simulink library "notificaStato"  (R2024b)
settings: Solver=VariableStepAuto  StartTime=0.0  StopTime=10.0  RelTol=1e-3
settings Model: Creator=mainuser  LastModifiedBy=mainuser

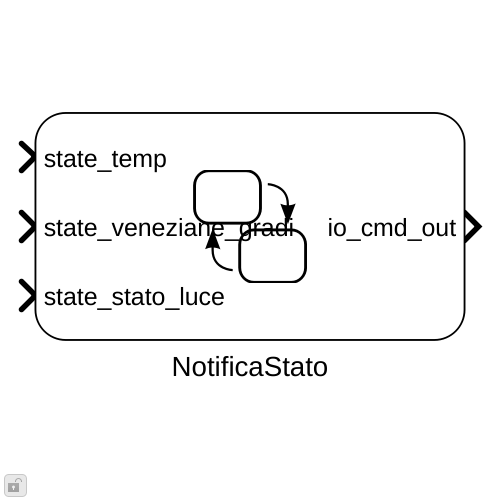
[thumbnail: Simulink's stored preview of the top-level diagram]
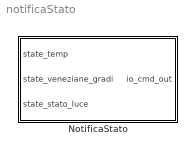
== system notificaStato ==
  NotificaStato : Stateflow chart  TreatAsAtomicUnit=on

== stateflow chart notificaStato/NotificaStato ==
  state SendNotify
    en: io_cmd_out = send_notifica(...
    state_temp, ...
    state_veneziane_gradi, ...
    state_stato_luce...
    )
  state Wait
  (default) -> SendNotify
  SendNotify -> Wait
  Wait -> SendNotify : after(10,sec)
  data: temp function_input uint8 size=1; angolo function_input uint8 size=1; stato_luce function_input boolean size=1; msgOut function_output string; state_temp input uint8 size=1; state_veneziane_gradi input uint8 size=1; state_stato_luce input boolean size=1; io_cmd_out output string
  function msgOut = send_notifica(temp, angolo, stato_luce):
    | function msgOut = send_notifica(temp, angolo, stato_luce)
    | % Crea una stringa di notifica sullo stato del sistema.
    | 
    | % Determina lo stato delle veneziane utilizzando un'istruzione switch.
    | switch angolo
    |     case 0
    |         stato_veneziane = 'chiuse';
    |     case 180
    |         stato_veneziane = 'aperte';
    |     otherwise
    |         stato_veneziane = sprintf('parzialmente aperte a %u grad', angolo);
    | end
    | 
    | % Determina lo stato delle luci (logica semplificata senza timer).
    | if stato_luce == false
    |     stato_luci = 'SPENTE';
    | else
    |     stato_luci = 'ACCESE';
    | end
    | 
    | % Compone il messaggio finale in un unico passaggio e lo converte in stringa.
    | msgOut = string(sprintf([...
    |     '\n=== STATO SISTEMA ===\n' ...
    |     'Temperatura: %u C\n' ...
    |     'Veneziane: %s\n' ...
    |     'Luci: %s\n' ...
    |     '===================\n'], ...
    |     temp, stato_veneziane, stato_luci));
    | end
